simulink model "cst_robotarm"  (R2023b)
settings: Solver=ode23t  StartTime=0.0  StopTime=5  FixedStep=0.0001  MaxStep=0.05  RelTol=1e-3  EnableMultiTasking=on
model workspace (MAT data in the model file):
  DCMotor_J = 0.0946866703633
  DCMotor_K = 0.477771340295
  DCMotor_Kf = 0.921434142151
  DCMotor_L = 0.000316454712175
  DCMotor_R = 4.99938152603
  Ts = 0.1
  dFilt = [1 -0.1202]
  nFilt = [0.4399 0.4399]
values from neighbouring files (symbols this model uses):
  Kd = params(3)    [PIDOptimizer.m]    (also in Pid_DIff_Evol_3.m = x(3); cost.m = param(3); cost_adapted.m = param(3); cost_adopted.m = param(3))
  Ki = params(2)    [PIDOptimizer.m]    (also in Pid_DIff_Evol_3.m = x(2); cost.m = param(2); cost_adapted.m = param(2); cost_adopted.m = param(2))
  Kp = params(1)    [PIDOptimizer.m]    (also in Pid_DIff_Evol_3.m = x(1); cost.m = param(1); cost_adapted.m = param(1); cost_adopted.m = param(1))
  m = s(1)    [PIDOptimizer.m]    (also in cost.m; cost_adapted.m; cost_adopted.m)
  s = size(signals)    [PIDOptimizer.m]    (also in cost.m; cost_adapted.m; cost_adopted.m)
undefined symbols (not defined in the file or in its folder): joint1_ctrl, joint2_ctrl, joint3_ctrl, joint4_ctrl, joint5_ctrl, joint6_ctrl, X, Y, Z
libraries: sm_lib x244, fl_lib x75, nesl_utility x28, ee_lib x21, slpidlib x6, SignalEditorBlockLib x1
(part 7 of 7)

== system cst_robotarm/6 DOF Robot Arm/DC Motors/Turntable Motor/Power Amplifier/SL2Vbrk ==
  Signal : Inport
  Electrical Reference1 : fl_lib/Electrical/Electrical Elements/Electrical Reference
  Simulink to Physical Signal1 : nesl_utility/Simulink-PS Converter  PhysicalDomain=network_engine_domain  SubClassName=ps_input  LeftPortType=input  RightPortType=output  PseudoPeriodic=off  Frequencies=[]  NoiseDistribution=none  NoiseParameters=[]  Unit=V  AffineConversion=off  FilteringAndDerivatives=zero  SimscapeFilterOrder=1  InputFilterTimeConstant=.001  UdotUserProvided=0
  Voltage Source : fl_lib/Electrical/Electrical Sources/Controlled Voltage Source
  Volts : PMIOPort  Tag=PMCPort  Side=Right
  wires:
  Signal/1 -> Simulink to Physical Signal1/1
  connections:
  Voltage Source/LConn1 -- Volts/RConn1
  Simulink to Physical Signal1/RConn1 -- Voltage Source/RConn1
  Electrical Reference1/LConn1 -- Voltage Source/RConn2

== system cst_robotarm/6 DOF Robot Arm/DC Motors/Turntable Motor/Power Amplifier/SL2Vduty ==
  Signal : Inport
  Electrical Reference1 : fl_lib/Electrical/Electrical Elements/Electrical Reference
  Simulink to Physical Signal1 : nesl_utility/Simulink-PS Converter  PhysicalDomain=network_engine_domain  SubClassName=ps_input  LeftPortType=input  RightPortType=output  PseudoPeriodic=off  Frequencies=[]  NoiseDistribution=none  NoiseParameters=[]  Unit=V  AffineConversion=off  FilteringAndDerivatives=zero  SimscapeFilterOrder=1  InputFilterTimeConstant=.001  UdotUserProvided=0
  Voltage Source : fl_lib/Electrical/Electrical Sources/Controlled Voltage Source
  Volts : PMIOPort  Tag=PMCPort  Side=Right
  wires:
  Signal/1 -> Simulink to Physical Signal1/1
  connections:
  Voltage Source/LConn1 -- Volts/RConn1
  Simulink to Physical Signal1/RConn1 -- Voltage Source/RConn1
  Electrical Reference1/LConn1 -- Voltage Source/RConn2

== system cst_robotarm/6 DOF Robot Arm/DC Motors/Turntable Motor/Power Amplifier/SL2Vrev ==
  Signal : Inport
  Electrical Reference1 : fl_lib/Electrical/Electrical Elements/Electrical Reference
  Simulink to Physical Signal1 : nesl_utility/Simulink-PS Converter  PhysicalDomain=network_engine_domain  SubClassName=ps_input  LeftPortType=input  RightPortType=output  PseudoPeriodic=off  Frequencies=[]  NoiseDistribution=none  NoiseParameters=[]  Unit=V  AffineConversion=off  FilteringAndDerivatives=zero  SimscapeFilterOrder=1  InputFilterTimeConstant=.001  UdotUserProvided=0
  Voltage Source : fl_lib/Electrical/Electrical Sources/Controlled Voltage Source
  Volts : PMIOPort  Tag=PMCPort  Side=Right
  wires:
  Signal/1 -> Simulink to Physical Signal1/1
  connections:
  Electrical Reference1/LConn1 -- Voltage Source/RConn2
  Simulink to Physical Signal1/RConn1 -- Voltage Source/RConn1
  Voltage Source/LConn1 -- Volts/RConn1

== system cst_robotarm/6 DOF Robot Arm/DC Motors/Wrist Motor/Power Amplifier/SL2Vbrk ==
  Signal : Inport
  Electrical Reference1 : fl_lib/Electrical/Electrical Elements/Electrical Reference
  Simulink to Physical Signal1 : nesl_utility/Simulink-PS Converter  PhysicalDomain=network_engine_domain  SubClassName=ps_input  LeftPortType=input  RightPortType=output  PseudoPeriodic=off  Frequencies=[]  NoiseDistribution=none  NoiseParameters=[]  Unit=V  AffineConversion=off  FilteringAndDerivatives=zero  SimscapeFilterOrder=1  InputFilterTimeConstant=.001  UdotUserProvided=0
  Voltage Source : fl_lib/Electrical/Electrical Sources/Controlled Voltage Source
  Volts : PMIOPort  Tag=PMCPort  Side=Right
  wires:
  Signal/1 -> Simulink to Physical Signal1/1
  connections:
  Electrical Reference1/LConn1 -- Voltage Source/RConn2
  Simulink to Physical Signal1/RConn1 -- Voltage Source/RConn1
  Voltage Source/LConn1 -- Volts/RConn1

== system cst_robotarm/6 DOF Robot Arm/DC Motors/Wrist Motor/Power Amplifier/SL2Vduty ==
  Signal : Inport
  Electrical Reference1 : fl_lib/Electrical/Electrical Elements/Electrical Reference
  Simulink to Physical Signal1 : nesl_utility/Simulink-PS Converter  PhysicalDomain=network_engine_domain  SubClassName=ps_input  LeftPortType=input  RightPortType=output  PseudoPeriodic=off  Frequencies=[]  NoiseDistribution=none  NoiseParameters=[]  Unit=V  AffineConversion=off  FilteringAndDerivatives=zero  SimscapeFilterOrder=1  InputFilterTimeConstant=.001  UdotUserProvided=0
  Voltage Source : fl_lib/Electrical/Electrical Sources/Controlled Voltage Source
  Volts : PMIOPort  Tag=PMCPort  Side=Right
  wires:
  Signal/1 -> Simulink to Physical Signal1/1
  connections:
  Electrical Reference1/LConn1 -- Voltage Source/RConn2
  Simulink to Physical Signal1/RConn1 -- Voltage Source/RConn1
  Voltage Source/LConn1 -- Volts/RConn1

== system cst_robotarm/6 DOF Robot Arm/DC Motors/Wrist Motor/Power Amplifier/SL2Vrev ==
  Signal : Inport
  Electrical Reference1 : fl_lib/Electrical/Electrical Elements/Electrical Reference
  Simulink to Physical Signal1 : nesl_utility/Simulink-PS Converter  PhysicalDomain=network_engine_domain  SubClassName=ps_input  LeftPortType=input  RightPortType=output  PseudoPeriodic=off  Frequencies=[]  NoiseDistribution=none  NoiseParameters=[]  Unit=V  AffineConversion=off  FilteringAndDerivatives=zero  SimscapeFilterOrder=1  InputFilterTimeConstant=.001  UdotUserProvided=0
  Voltage Source : fl_lib/Electrical/Electrical Sources/Controlled Voltage Source
  Volts : PMIOPort  Tag=PMCPort  Side=Right
  wires:
  Signal/1 -> Simulink to Physical Signal1/1
  connections:
  Voltage Source/LConn1 -- Volts/RConn1
  Simulink to Physical Signal1/RConn1 -- Voltage Source/RConn1
  Electrical Reference1/LConn1 -- Voltage Source/RConn2

== system cst_robotarm/6 DOF Robot Arm/6 DOF Robot Arm Mechanics/Wrist/MotorWristAsm_1_RIGID/ServoTJD2_1_RIGID/bottom_cover_1_RIGID ==
  ReferenceFrame : sm_lib/Frames and Transforms/Reference Frame
  Solid : sm_lib/Body Elements/File Solid  ExtGeomFileName=bottomCover_Default_sldprt.STL  UnitType=Custom  ExtGeomFileUnits=mm  StepReaderType=HEX  ExportConvexHullGeometry=off  InertiaType=Custom  Mass=0.0069725116500885713  MassUnits=kg  CenterOfMass=[0 0.85958385692466177 0]  CenterOfMassUnits=mm  MomentsOfInertia=[0.21879995145338263 1.0303249150901777 0.81533794134290127]  MomentsOfInertiaUnits=kg*mm^2  ProductsOfInertia=[0 0 0]  ProductsOfInertiaUnits=kg*mm^2  BasedOnType=Density  Density=1000  DensityUnits=kg/(m^3)  DoExposeReferenceFrame=on  SerializedFrames=<Frames/>  GraphicType=FromGeometry  MarkerShape=Sphere  MarkerSize=10  MarkerSizeUnits=m  GraphicVisPropType=SimpleVisualProperties  GraphicDiffuseColor=[0.4 0.4 0.4]  GraphicSpecularColor=[0.5 0.5 0.5 1.0]  GraphicAmbientColor=[0.15 0.15 0.15 1.0]  GraphicEmissiveColor=[0.0 0.0 0.0 1.0]  GraphicShininess=75  GraphicOpacity=1
  F : PMIOPort  Side=Left
  connections:
  Solid/RConn1 -- ReferenceFrame/RConn1 -- F/RConn1

== system cst_robotarm/6 DOF Robot Arm/6 DOF Robot Arm Mechanics/Wrist/MotorWristAsm_1_RIGID/ServoTJD2_1_RIGID/servo_Case_1_RIGID ==
  ReferenceFrame : sm_lib/Frames and Transforms/Reference Frame
  Solid : sm_lib/Body Elements/File Solid  ExtGeomFileName=servoCase_Default_sldprt.STL  UnitType=Custom  ExtGeomFileUnits=mm  StepReaderType=HEX  ExportConvexHullGeometry=off  InertiaType=Custom  Mass=0.024788567791665928  MassUnits=kg  CenterOfMass=[0.08042125391634411 -6.0857711413150408 -0.045303315504018803]  CenterOfMassUnits=mm  MomentsOfInertia=[2.4475554038950817 5.416405903149534 5.3480430794560796]  MomentsOfInertiaUnits=kg*mm^2  ProductsOfInertia=[0.0035757453477574665 0.0080258931443943603 -0.048088274914116991]  ProductsOfInertiaUnits=kg*mm^2  BasedOnType=Density  Density=1000  DensityUnits=kg/(m^3)  DoExposeReferenceFrame=on  SerializedFrames=<Frames/>  GraphicType=FromGeometry  MarkerShape=Sphere  MarkerSize=10  MarkerSizeUnits=m  GraphicVisPropType=SimpleVisualProperties  GraphicDiffuseColor=[0.4 0.4 0.4]  GraphicSpecularColor=[0.5 0.5 0.5 1.0]  GraphicAmbientColor=[0.15 0.15 0.15 1.0]  GraphicEmissiveColor=[0.0 0.0 0.0 1.0]  GraphicShininess=75  GraphicOpacity=1
  F : PMIOPort  Side=Left
  connections:
  Solid/RConn1 -- ReferenceFrame/RConn1 -- F/RConn1

== system cst_robotarm/6 DOF Robot Arm/6 DOF Robot Arm Mechanics/Wrist/MotorWristAsm_1_RIGID/ServoTJD2_1_RIGID/servo_cover_2_RIGID ==
  ReferenceFrame : sm_lib/Frames and Transforms/Reference Frame
  Solid : sm_lib/Body Elements/File Solid  ExtGeomFileName=servoCover_Default_sldprt.STL  UnitType=Custom  ExtGeomFileUnits=mm  StepReaderType=HEX  ExportConvexHullGeometry=off  InertiaType=Custom  Mass=0.018198073455255783  MassUnits=kg  CenterOfMass=[19.173079671185903 9.8425000000000011 6.6069555093490839]  CenterOfMassUnits=mm  MomentsOfInertia=[1.0514460019053871 4.1870037592553642 4.7863110501402781]  MomentsOfInertiaUnits=kg*mm^2  ProductsOfInertia=[0 0.046415809435786888 0]  ProductsOfInertiaUnits=kg*mm^2  BasedOnType=Density  Density=1000  DensityUnits=kg/(m^3)  DoExposeReferenceFrame=on  SerializedFrames=<Frames/>  GraphicType=FromGeometry  MarkerShape=Sphere  MarkerSize=10  MarkerSizeUnits=m  GraphicVisPropType=SimpleVisualProperties  GraphicDiffuseColor=[0.6 0.6 0.6]  GraphicSpecularColor=[0.5 0.5 0.5 1.0]  GraphicAmbientColor=[0.15 0.15 0.15 1.0]  GraphicEmissiveColor=[0.0 0.0 0.0 1.0]  GraphicShininess=75  GraphicOpacity=1
  F : PMIOPort  Side=Left
  connections:
  Solid/RConn1 -- ReferenceFrame/RConn1 -- F/RConn1
